simulink model "tp3_sys_asserv_schema"  (R2014a)
settings: Solver=ode45  SolverMode=SingleTasking  StartTime=0.0  StopTime=100  RelTol=1e-3
undefined symbols (not defined in the file or in its folder): k1, k2, Te
settings Model: Creator=e12108993  LastModifiedBy=UTILISATEUR
settings OptimizationCC: BlockReduction=off  BooleanDataType=off
settings DebuggingCC: SaveWithParameterizedLinksMsg=none  UnderspecifiedInitializationDetection=Classic  SignalResolutionControl=TryResolveAllWithWarning  SolverPrmCheckMsg=none
settings HardwareCC: TargetUnknown=on

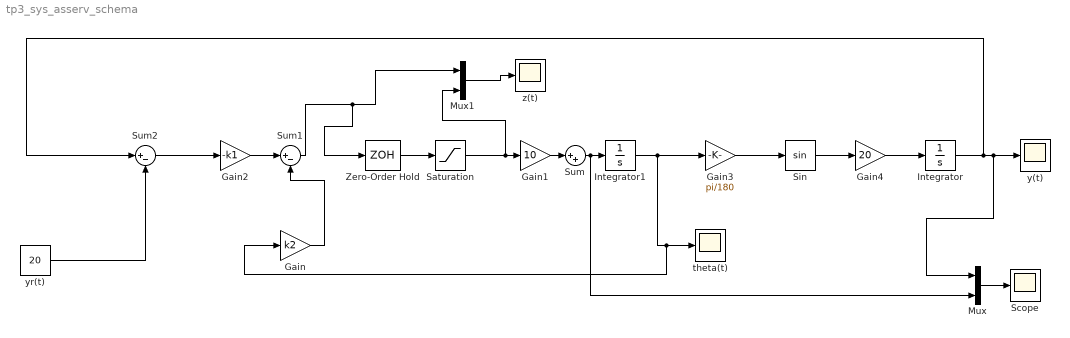
== system tp3_sys_asserv_schema ==
  Gain : Gain  Gain=k2
  Gain1 : Gain  Gain=10
  Gain2 : Gain  Gain=-k1
  Gain3 : Gain  Gain=pi/180
  Gain4 : Gain  Gain=20
  Integrator : Integrator
  Integrator1 : Integrator
  Mux : Mux  Inputs=2
  Mux1 : Mux  Inputs=2
  Saturation : Saturate  UpperLimit=10  LowerLimit=-10
  Scope : Scope
  Sin : Trigonometry
  Sum : Sum  Inputs=|++
  Sum1 : Sum  Inputs=|+-
  Sum2 : Sum  Inputs=|+-
  Zero-Order Hold : ZeroOrderHold  SampleTime=Te
  theta(t) : Scope
  "y(t) " : Scope
  "yr(t) " : Constant  Value=20
  "z(t) " : Scope
  wires:
  "yr(t) "/1 -> Sum2/2
  Sum2/1 -> Gain2/1
  Gain2/1 -> Sum1/1
  Gain/1 -> Sum1/2
  Sum1/1 -> Mux1/1, Zero-Order Hold/1
  Sum/1 -> Mux/2, Integrator1/1
  Integrator1/1 -> Gain3/1, theta(t)/1, Gain/1
  Gain3/1 -> Sin/1
  Sin/1 -> Gain4/1
  Gain4/1 -> Integrator/1
  Integrator/1 -> Sum2/1, Mux/1, "y(t) "/1
  Mux/1 -> Scope/1
  Mux1/1 -> "z(t) "/1
  Zero-Order Hold/1 -> Saturation/1
  Saturation/1 -> Mux1/2, Gain1/1
  Gain1/1 -> Sum/1
